simulink model "MSBR_Plant"  (R2021b)
settings: Solver=ode45  StartTime=0.0  StopTime=sim_time  MaxStep=ts_max  RelTol=1e-4
values from neighbouring files (symbols this model uses):
  a_1 = 8.7292e-2/wilson_ratio    (= 0.0087292)    [Whole_Plant_Cool_Pump_Accident_script.m]    (also in Whole_Plant_Fert_Pump_Accident_script.m; Whole_Plant_Fuel_Pump_Accident.m; Whole_Plant_Fuel_Pump_Accident_script.m; Whole_Plant_Reactivity_Accident.m)
  a_2 = 7.3787e-4/wilson_ratio    (= 7.3787e-05)    [Whole_Plant_Cool_Pump_Accident_script.m]    (also in Whole_Plant_Fert_Pump_Accident_script.m; Whole_Plant_Fuel_Pump_Accident.m; Whole_Plant_Fuel_Pump_Accident_script.m; Whole_Plant_Reactivity_Accident.m)
  a_b = 1.656e-5    (= 1.656e-05)    [Whole_Plant_Cool_Pump_Accident_script.m]    (also in Whole_Plant_Fert_Pump_Accident_script.m; Whole_Plant_Fuel_Pump_Accident.m; Whole_Plant_Fuel_Pump_Accident_script.m; Whole_Plant_Reactivity_Accident.m)
  a_f = -8.172e-5    (= -8.172e-05)    [Whole_Plant_Cool_Pump_Accident_script.m]    (also in Whole_Plant_Fert_Pump_Accident_script.m; Whole_Plant_Fuel_Pump_Accident.m; Whole_Plant_Fuel_Pump_Accident_script.m; Whole_Plant_Reactivity_Accident.m)
  a_g = 2.016e-5    (= 2.016e-05)    [Whole_Plant_Cool_Pump_Accident_script.m]    (also in Whole_Plant_Fert_Pump_Accident_script.m; Whole_Plant_Fuel_Pump_Accident.m; Whole_Plant_Fuel_Pump_Accident_script.m; Whole_Plant_Reactivity_Accident.m)
  A_s = pi()*((D_OTSG_i^2)/4) - A_w_OTSG - A_p_OTSG    [Whole_Plant_Cool_Pump_Accident_script.m]    (also in Whole_Plant_Fert_Pump_Accident_script.m; Whole_Plant_Fuel_Pump_Accident.m; Whole_Plant_Fuel_Pump_Accident_script.m; Whole_Plant_Reactivity_Accident.m)
  alpha_co = 316.2    [Whole_Plant_Cool_Pump_Accident_script.m]    (also in Whole_Plant_Fert_Pump_Accident_script.m; Whole_Plant_Fuel_Pump_Accident.m; Whole_Plant_Fuel_Pump_Accident_script.m; Whole_Plant_Reactivity_Accident.m)
  beta = [2.290e-04, 8.320e-04, 7.100e-04, 8.520e-04, 1.710e-04, 1.020e-04]    [Whole_Plant_Cool_Pump_Accident_script.m]    (also in Whole_Plant_Fert_Pump_Accident_script.m; Whole_Plant_Fuel_Pump_Accident.m; Whole_Plant_Fuel_Pump_Accident_script.m; Whole_Plant_Reactivity_Accident.m)
  beta_co = 68.0958    [Whole_Plant_Cool_Pump_Accident_script.m]    (also in Whole_Plant_Fert_Pump_Accident_script.m; Whole_Plant_Fuel_Pump_Accident.m; Whole_Plant_Fuel_Pump_Accident_script.m; Whole_Plant_Reactivity_Accident.m)
  beta_t = sum(beta)    [Whole_Plant_Cool_Pump_Accident_script.m]    (also in Whole_Plant_Fert_Pump_Accident_script.m; Whole_Plant_Fuel_Pump_Accident.m; Whole_Plant_Fuel_Pump_Accident_script.m; Whole_Plant_Reactivity_Accident.m)
  C_nc_X_A_nc = 12.8    [Whole_Plant_Cool_Pump_Accident_script.m]    (also in Whole_Plant_Fert_Pump_Accident_script.m; Whole_Plant_Fuel_Pump_Accident.m; Whole_Plant_Fuel_Pump_Accident_script.m; Whole_Plant_Reactivity_Accident.m)
  C_pcw = 0.0042    [Whole_Plant_Cool_Pump_Accident_script.m]    (also in Whole_Plant_Fert_Pump_Accident_script.m; Whole_Plant_Fuel_Pump_Accident.m; Whole_Plant_Fuel_Pump_Accident_script.m; Whole_Plant_Reactivity_Accident.m)
  C_rh_X_A_rh = 33    [Whole_Plant_Cool_Pump_Accident_script.m]    (also in Whole_Plant_Fert_Pump_Accident_script.m; Whole_Plant_Fuel_Pump_Accident.m; Whole_Plant_Fuel_Pump_Accident_script.m; Whole_Plant_Reactivity_Accident.m)
  C_v = 0.84    [Whole_Plant_Cool_Pump_Accident_script.m]    (also in Whole_Plant_Fert_Pump_Accident_script.m; Whole_Plant_Fuel_Pump_Accident.m; Whole_Plant_Fuel_Pump_Accident_script.m; Whole_Plant_Reactivity_Accident.m)
  ce1 = 1.2471e-07    [Whole_Plant_Cool_Pump_Accident_script.m]    (also in Whole_Plant_Fert_Pump_Accident_script.m; Whole_Plant_Fuel_Pump_Accident.m; Whole_Plant_Fuel_Pump_Accident_script.m; Whole_Plant_Reactivity_Accident.m)
  ce2 = 5.3816e-14    [Whole_Plant_Cool_Pump_Accident_script.m]    (also in Whole_Plant_Fert_Pump_Accident_script.m; Whole_Plant_Fuel_Pump_Accident.m; Whole_Plant_Fuel_Pump_Accident_script.m; Whole_Plant_Reactivity_Accident.m)
  ce3 = 3.3721e-08    [Whole_Plant_Cool_Pump_Accident_script.m]    (also in Whole_Plant_Fert_Pump_Accident_script.m; Whole_Plant_Fuel_Pump_Accident.m; Whole_Plant_Fuel_Pump_Accident_script.m; Whole_Plant_Reactivity_Accident.m)
  Cp_fw = XSteam('Cp_pT',P_set*10,T_fw)/1000    [Whole_Plant_Cool_Pump_Accident_script.m]    (also in Whole_Plant_Fert_Pump_Accident_script.m; Whole_Plant_Fuel_Pump_Accident.m; Whole_Plant_Fuel_Pump_Accident_script.m; Whole_Plant_Reactivity_Accident.m)
  Cp_p = Cp_sec    (= 0.001716588)    [Whole_Plant_Cool_Pump_Accident_script.m]    (also in Whole_Plant_Fert_Pump_Accident_script.m; Whole_Plant_Fuel_Pump_Accident.m; Whole_Plant_Fuel_Pump_Accident_script.m; Whole_Plant_Reactivity_Accident.m)
  Cp_rh = 0.0021520    (= 0.002152)    [Whole_Plant_Cool_Pump_Accident_script.m]    (also in Whole_Plant_Fert_Pump_Accident_script.m; Whole_Plant_Fuel_Pump_Accident.m; Whole_Plant_Fuel_Pump_Accident_script.m; Whole_Plant_Reactivity_Accident.m)
  Cp_s = XSteam('Cp_pT',P_s*10,T_s)/1000    [Whole_Plant_Cool_Pump_Accident_script.m]    (also in Whole_Plant_Fert_Pump_Accident_script.m; Whole_Plant_Fuel_Pump_Accident.m; Whole_Plant_Fuel_Pump_Accident_script.m; Whole_Plant_Reactivity_Accident.m)
  Cp_sc = XSteam('Cp_pT',P_set*10,T_sc2)/1000    [Whole_Plant_Cool_Pump_Accident_script.m]    (also in Whole_Plant_Fert_Pump_Accident_script.m; Whole_Plant_Fuel_Pump_Accident.m; Whole_Plant_Fuel_Pump_Accident_script.m; Whole_Plant_Reactivity_Accident.m)
  Cp_w = 468.992e-6    (= 0.000468992)    [Whole_Plant_Cool_Pump_Accident_script.m]    (also in Whole_Plant_Fert_Pump_Accident_script.m; Whole_Plant_Fuel_Pump_Accident.m; Whole_Plant_Fuel_Pump_Accident_script.m; Whole_Plant_Reactivity_Accident.m)
  D_it = D_ot-2*T_th    (= 0.014147)    [Whole_Plant_Cool_Pump_Accident_script.m]    (also in Whole_Plant_Fert_Pump_Accident_script.m; Whole_Plant_Fuel_Pump_Accident.m; Whole_Plant_Fuel_Pump_Accident_script.m; Whole_Plant_Reactivity_Accident.m)
  D_ot = 0.015875    [Whole_Plant_Cool_Pump_Accident_script.m]    (also in Whole_Plant_Fert_Pump_Accident_script.m; Whole_Plant_Fuel_Pump_Accident.m; Whole_Plant_Fuel_Pump_Accident_script.m; Whole_Plant_Reactivity_Accident.m)
  dHs_dPs = c(1)    [Whole_Plant_Cool_Pump_Accident_script.m]    (also in Whole_Plant_Fert_Pump_Accident_script.m; Whole_Plant_Fuel_Pump_Accident.m; Whole_Plant_Fuel_Pump_Accident_script.m; Whole_Plant_Reactivity_Accident.m)
  eta_hp_isen = 0.861    [Whole_Plant_Cool_Pump_Accident_script.m]    (also in Whole_Plant_Fert_Pump_Accident_script.m; Whole_Plant_Fuel_Pump_Accident.m; Whole_Plant_Fuel_Pump_Accident_script.m; Whole_Plant_Reactivity_Accident.m)
  eta_lp_isen = 0.861    [Whole_Plant_Cool_Pump_Accident_script.m]    (also in Whole_Plant_Fert_Pump_Accident_script.m; Whole_Plant_Fuel_Pump_Accident.m; Whole_Plant_Fuel_Pump_Accident_script.m; Whole_Plant_Reactivity_Accident.m)
  gamma_I = 5.1135e-2    (= 0.051135)    [Whole_Plant_Cool_Pump_Accident_script.m]    (also in Whole_Plant_Fert_Pump_Accident_script.m; Whole_Plant_Fuel_Pump_Accident.m; Whole_Plant_Fuel_Pump_Accident_script.m; Whole_Plant_Reactivity_Accident.m)
  gamma_Xe = 1.1628e-2    (= 0.011628)    [Whole_Plant_Cool_Pump_Accident_script.m]    (also in Whole_Plant_Fert_Pump_Accident_script.m; Whole_Plant_Fuel_Pump_Accident.m; Whole_Plant_Fuel_Pump_Accident_script.m; Whole_Plant_Reactivity_Accident.m)
  H_co0 = 0.149    [Whole_Plant_Cool_Pump_Accident_script.m]    (also in Whole_Plant_Fert_Pump_Accident_script.m; Whole_Plant_Fuel_Pump_Accident.m; Whole_Plant_Fuel_Pump_Accident_script.m; Whole_Plant_Reactivity_Accident.m)
  H_f_co0 = 0.149    [Whole_Plant_Cool_Pump_Accident_script.m]    (also in Whole_Plant_Fert_Pump_Accident_script.m; Whole_Plant_Fuel_Pump_Accident.m; Whole_Plant_Fuel_Pump_Accident_script.m; Whole_Plant_Reactivity_Accident.m)
  H_fg_co0 = 2.35    [Whole_Plant_Cool_Pump_Accident_script.m]    (also in Whole_Plant_Fert_Pump_Accident_script.m; Whole_Plant_Fuel_Pump_Accident.m; Whole_Plant_Fuel_Pump_Accident_script.m; Whole_Plant_Reactivity_Accident.m)
  H_fgrh0 = (XSteam('hV_p', P_s*1e1) - XSteam('hL_p', P_s*1e1))/1e3    [Whole_Plant_Cool_Pump_Accident_script.m]    (also in Whole_Plant_Fert_Pump_Accident_script.m; Whole_Plant_Fuel_Pump_Accident.m; Whole_Plant_Fuel_Pump_Accident_script.m; Whole_Plant_Reactivity_Accident.m)
  H_frh0 = XSteam('hL_p', P_s*1e1)/1e3    [Whole_Plant_Cool_Pump_Accident_script.m]    (also in Whole_Plant_Fert_Pump_Accident_script.m; Whole_Plant_Fuel_Pump_Accident.m; Whole_Plant_Fuel_Pump_Accident_script.m; Whole_Plant_Reactivity_Accident.m)
  h_fwh1 = 0.5927    [Whole_Plant_Cool_Pump_Accident_script.m]    (also in Whole_Plant_Fert_Pump_Accident_script.m; Whole_Plant_Fuel_Pump_Accident.m; Whole_Plant_Fuel_Pump_Accident_script.m; Whole_Plant_Reactivity_Accident.m)
  H_fwh10 = 0.46009    [Whole_Plant_Cool_Pump_Accident_script.m]    (also in Whole_Plant_Fert_Pump_Accident_script.m; Whole_Plant_Fuel_Pump_Accident.m; Whole_Plant_Fuel_Pump_Accident_script.m; Whole_Plant_Reactivity_Accident.m)
  h_fwh2 = 1.230803    [Whole_Plant_Cool_Pump_Accident_script.m]    (also in Whole_Plant_Fert_Pump_Accident_script.m; Whole_Plant_Fuel_Pump_Accident.m; Whole_Plant_Fuel_Pump_Accident_script.m; Whole_Plant_Reactivity_Accident.m)
  H_fwh20 = 0.6784    [Whole_Plant_Cool_Pump_Accident_script.m]    (also in Whole_Plant_Fert_Pump_Accident_script.m; Whole_Plant_Fuel_Pump_Accident.m; Whole_Plant_Fuel_Pump_Accident_script.m; Whole_Plant_Reactivity_Accident.m)
  H_grh0 = 2.8029    [Whole_Plant_Cool_Pump_Accident_script.m]    (also in Whole_Plant_Fert_Pump_Accident_script.m; Whole_Plant_Fuel_Pump_Accident.m; Whole_Plant_Fuel_Pump_Accident_script.m; Whole_Plant_Reactivity_Accident.m)
  H_hp_isen0 = 2.5111    [Whole_Plant_Cool_Pump_Accident_script.m]    (also in Whole_Plant_Fert_Pump_Accident_script.m; Whole_Plant_Fuel_Pump_Accident.m; Whole_Plant_Fuel_Pump_Accident_script.m; Whole_Plant_Reactivity_Accident.m)
  H_hpt_out = 2.6201    [Whole_Plant_Cool_Pump_Accident_script.m]    (also in Whole_Plant_Fert_Pump_Accident_script.m; Whole_Plant_Fuel_Pump_Accident.m; Whole_Plant_Fuel_Pump_Accident_script.m; Whole_Plant_Reactivity_Accident.m)
  H_lp_isen = 958.4*1054.35e-6/0.45359237    (= 2.22774699671)    [Whole_Plant_Cool_Pump_Accident_script.m]    (also in Whole_Plant_Fert_Pump_Accident_script.m; Whole_Plant_Fuel_Pump_Accident.m; Whole_Plant_Fuel_Pump_Accident_script.m; Whole_Plant_Reactivity_Accident.m)
  H_lpt_out = 2.3089    [Whole_Plant_Cool_Pump_Accident_script.m]    (also in Whole_Plant_Fert_Pump_Accident_script.m; Whole_Plant_Fuel_Pump_Accident.m; Whole_Plant_Fuel_Pump_Accident_script.m; Whole_Plant_Reactivity_Accident.m)
  H_nc = XSteam('h_pT', P_s*10, T_s)/1000    [Whole_Plant_Cool_Pump_Accident_script.m]    (also in Whole_Plant_Fert_Pump_Accident_script.m; Whole_Plant_Fuel_Pump_Accident.m; Whole_Plant_Fuel_Pump_Accident_script.m; Whole_Plant_Reactivity_Accident.m)
  h_pw = h_s    (= 0.02555)    [Whole_Plant_Cool_Pump_Accident_script.m]    (also in Whole_Plant_Fert_Pump_Accident_script.m; Whole_Plant_Fuel_Pump_Accident.m; Whole_Plant_Fuel_Pump_Accident_script.m; Whole_Plant_Reactivity_Accident.m)
  H_rh = 2.8115    [Whole_Plant_Cool_Pump_Accident_script.m]    (also in Whole_Plant_Fert_Pump_Accident_script.m; Whole_Plant_Fuel_Pump_Accident.m; Whole_Plant_Fuel_Pump_Accident_script.m; Whole_Plant_Reactivity_Accident.m)
  h_wb = 13349.334646671E-6    (= 0.0133493346467)    [Whole_Plant_Cool_Pump_Accident_script.m]    (also in Whole_Plant_Fert_Pump_Accident_script.m; Whole_Plant_Fuel_Pump_Accident.m; Whole_Plant_Fuel_Pump_Accident_script.m; Whole_Plant_Reactivity_Accident.m)
  h_ws = 5732.378387768E-6    (= 0.00573237838777)    [Whole_Plant_Cool_Pump_Accident_script.m]    (also in Whole_Plant_Fert_Pump_Accident_script.m; Whole_Plant_Fuel_Pump_Accident.m; Whole_Plant_Fuel_Pump_Accident_script.m; Whole_Plant_Reactivity_Accident.m)
  h_wsc = 8385.005556375E-6    (= 0.00838500555638)    [Whole_Plant_Cool_Pump_Accident_script.m]    (also in Whole_Plant_Fert_Pump_Accident_script.m; Whole_Plant_Fuel_Pump_Accident.m; Whole_Plant_Fuel_Pump_Accident_script.m; Whole_Plant_Reactivity_Accident.m)
  hA_bg = A_fert*h_bg    (= 2.76411813627)    [Whole_Plant_Cool_Pump_Accident_script.m]    (also in Whole_Plant_Fert_Pump_Accident_script.m; Whole_Plant_Fuel_Pump_Accident.m; Whole_Plant_Fuel_Pump_Accident_script.m; Whole_Plant_Reactivity_Accident.m)
  hA_co0 = 140    [Whole_Plant_Cool_Pump_Accident_script.m]    (also in Whole_Plant_Fert_Pump_Accident_script.m; Whole_Plant_Fuel_Pump_Accident.m; Whole_Plant_Fuel_Pump_Accident_script.m; Whole_Plant_Reactivity_Accident.m)
  hA_fg_dn = h_fg*A_fuel_down    [Whole_Plant_Cool_Pump_Accident_script.m]    (also in Whole_Plant_Fert_Pump_Accident_script.m; Whole_Plant_Fuel_Pump_Accident.m; Whole_Plant_Fuel_Pump_Accident_script.m; Whole_Plant_Reactivity_Accident.m)
  hA_fg_up = h_fg*A_fuel_up    [Whole_Plant_Cool_Pump_Accident_script.m]    (also in Whole_Plant_Fert_Pump_Accident_script.m; Whole_Plant_Fuel_Pump_Accident.m; Whole_Plant_Fuel_Pump_Accident_script.m; Whole_Plant_Reactivity_Accident.m)
  hA_p_bhx1 = [h_pb*A_pbhx/2,h_pb*A_pbhx/2]    [Whole_Plant_Cool_Pump_Accident_script.m]    (also in Whole_Plant_Fert_Pump_Accident_script.m; Whole_Plant_Fuel_Pump_Accident.m; Whole_Plant_Fuel_Pump_Accident_script.m; Whole_Plant_Reactivity_Accident.m)
  hA_p_bhx2 = hA_p_bhx1    [Whole_Plant_Cool_Pump_Accident_script.m]    (also in Whole_Plant_Fert_Pump_Accident_script.m; Whole_Plant_Fuel_Pump_Accident.m; Whole_Plant_Fuel_Pump_Accident_script.m; Whole_Plant_Reactivity_Accident.m)
  hA_p_bhx3 = hA_p_bhx1    [Whole_Plant_Cool_Pump_Accident_script.m]    (also in Whole_Plant_Fert_Pump_Accident_script.m; Whole_Plant_Fuel_Pump_Accident.m; Whole_Plant_Fuel_Pump_Accident_script.m; Whole_Plant_Reactivity_Accident.m)
  hA_p_bhx4 = hA_p_bhx1    [Whole_Plant_Cool_Pump_Accident_script.m]    (also in Whole_Plant_Fert_Pump_Accident_script.m; Whole_Plant_Fuel_Pump_Accident.m; Whole_Plant_Fuel_Pump_Accident_script.m; Whole_Plant_Reactivity_Accident.m)
  hA_p_fhx1 = [h_p*A_pfhx_dn/2,h_p*A_pfhx_dn/2,h_p*A_pfhx_up/2,h_p*A_pfhx_up/2]    [Whole_Plant_Cool_Pump_Accident_script.m]    (also in Whole_Plant_Fert_Pump_Accident_script.m; Whole_Plant_Fuel_Pump_Accident.m; Whole_Plant_Fuel_Pump_Accident_script.m; Whole_Plant_Reactivity_Accident.m)
  hA_p_fhx2 = hA_p_fhx1    [Whole_Plant_Cool_Pump_Accident_script.m]    (also in Whole_Plant_Fert_Pump_Accident_script.m; Whole_Plant_Fuel_Pump_Accident.m; Whole_Plant_Fuel_Pump_Accident_script.m; Whole_Plant_Reactivity_Accident.m)
  hA_p_fhx3 = hA_p_fhx1    [Whole_Plant_Cool_Pump_Accident_script.m]    (also in Whole_Plant_Fert_Pump_Accident_script.m; Whole_Plant_Fuel_Pump_Accident.m; Whole_Plant_Fuel_Pump_Accident_script.m; Whole_Plant_Reactivity_Accident.m)
  hA_p_fhx4 = hA_p_fhx1    [Whole_Plant_Cool_Pump_Accident_script.m]    (also in Whole_Plant_Fert_Pump_Accident_script.m; Whole_Plant_Fuel_Pump_Accident.m; Whole_Plant_Fuel_Pump_Accident_script.m; Whole_Plant_Reactivity_Accident.m)
  hA_s_bhx1 = [h_sb*A_sbhx/2,h_sb*A_sbhx/2]    [Whole_Plant_Cool_Pump_Accident_script.m]    (also in Whole_Plant_Fert_Pump_Accident_script.m; Whole_Plant_Fuel_Pump_Accident.m; Whole_Plant_Fuel_Pump_Accident_script.m; Whole_Plant_Reactivity_Accident.m)
  hA_s_bhx2 = hA_s_bhx1    [Whole_Plant_Cool_Pump_Accident_script.m]    (also in Whole_Plant_Fert_Pump_Accident_script.m; Whole_Plant_Fuel_Pump_Accident.m; Whole_Plant_Fuel_Pump_Accident_script.m; Whole_Plant_Reactivity_Accident.m)
  hA_s_bhx3 = hA_s_bhx1    [Whole_Plant_Cool_Pump_Accident_script.m]    (also in Whole_Plant_Fert_Pump_Accident_script.m; Whole_Plant_Fuel_Pump_Accident.m; Whole_Plant_Fuel_Pump_Accident_script.m; Whole_Plant_Reactivity_Accident.m)
  hA_s_bhx4 = hA_s_bhx1    [Whole_Plant_Cool_Pump_Accident_script.m]    (also in Whole_Plant_Fert_Pump_Accident_script.m; Whole_Plant_Fuel_Pump_Accident.m; Whole_Plant_Fuel_Pump_Accident_script.m; Whole_Plant_Reactivity_Accident.m)
  hA_s_fhx1 = [h_s*A_sfhx_up/2,h_s*A_sfhx_up/2,h_s*A_sfhx_dn/2,h_s*A_sfhx_dn/2]    [Whole_Plant_Cool_Pump_Accident_script.m]    (also in Whole_Plant_Fert_Pump_Accident_script.m; Whole_Plant_Fuel_Pump_Accident.m; Whole_Plant_Fuel_Pump_Accident_script.m; Whole_Plant_Reactivity_Accident.m)
  hA_s_fhx2 = hA_s_fhx1    [Whole_Plant_Cool_Pump_Accident_script.m]    (also in Whole_Plant_Fert_Pump_Accident_script.m; Whole_Plant_Fuel_Pump_Accident.m; Whole_Plant_Fuel_Pump_Accident_script.m; Whole_Plant_Reactivity_Accident.m)
  hA_s_fhx3 = hA_s_fhx1    [Whole_Plant_Cool_Pump_Accident_script.m]    (also in Whole_Plant_Fert_Pump_Accident_script.m; Whole_Plant_Fuel_Pump_Accident.m; Whole_Plant_Fuel_Pump_Accident_script.m; Whole_Plant_Reactivity_Accident.m)
  hA_s_fhx4 = hA_s_fhx1    [Whole_Plant_Cool_Pump_Accident_script.m]    (also in Whole_Plant_Fert_Pump_Accident_script.m; Whole_Plant_Fuel_Pump_Accident.m; Whole_Plant_Fuel_Pump_Accident_script.m; Whole_Plant_Reactivity_Accident.m)
  I_0 = gamma_I*Sigma_f_msbr*phi_0/lam_I    (= 1.30000734126e+17)    [Whole_Plant_Cool_Pump_Accident_script.m]    (also in Whole_Plant_Fert_Pump_Accident_script.m; Whole_Plant_Fuel_Pump_Accident.m; Whole_Plant_Fuel_Pump_Accident_script.m; Whole_Plant_Reactivity_Accident.m)
  k_1 = 0.5    [Whole_Plant_Cool_Pump_Accident_script.m]    (also in Whole_Plant_Fert_Pump_Accident_script.m; Whole_Plant_Fuel_Pump_Accident.m; Whole_Plant_Fuel_Pump_Accident_script.m; Whole_Plant_Reactivity_Accident.m)
  K_1 = e(1)    [Whole_Plant_Cool_Pump_Accident_script.m]    (also in Whole_Plant_Fert_Pump_Accident_script.m; Whole_Plant_Fuel_Pump_Accident.m; Whole_Plant_Fuel_Pump_Accident_script.m; Whole_Plant_Reactivity_Accident.m)
  k_1b = 0.5    [Whole_Plant_Cool_Pump_Accident_script.m]    (also in Whole_Plant_Fert_Pump_Accident_script.m; Whole_Plant_Fuel_Pump_Accident.m; Whole_Plant_Fuel_Pump_Accident_script.m; Whole_Plant_Reactivity_Accident.m)
  k_2 = 0.5    [Whole_Plant_Cool_Pump_Accident_script.m]    (also in Whole_Plant_Fert_Pump_Accident_script.m; Whole_Plant_Fuel_Pump_Accident.m; Whole_Plant_Fuel_Pump_Accident_script.m; Whole_Plant_Reactivity_Accident.m)
  k_2b = 0.5    [Whole_Plant_Cool_Pump_Accident_script.m]    (also in Whole_Plant_Fert_Pump_Accident_script.m; Whole_Plant_Fuel_Pump_Accident.m; Whole_Plant_Fuel_Pump_Accident_script.m; Whole_Plant_Reactivity_Accident.m)
  k_3 = 0.5    [Whole_Plant_Cool_Pump_Accident_script.m]    (also in Whole_Plant_Fert_Pump_Accident_script.m; Whole_Plant_Fuel_Pump_Accident.m; Whole_Plant_Fuel_Pump_Accident_script.m; Whole_Plant_Reactivity_Accident.m)
  k_4 = 0.5    [Whole_Plant_Cool_Pump_Accident_script.m]    (also in Whole_Plant_Fert_Pump_Accident_script.m; Whole_Plant_Fuel_Pump_Accident.m; Whole_Plant_Fuel_Pump_Accident_script.m; Whole_Plant_Reactivity_Accident.m)
  K_4 = b(1)    [Whole_Plant_Cool_Pump_Accident_script.m]    (also in Whole_Plant_Fert_Pump_Accident_script.m; Whole_Plant_Fuel_Pump_Accident.m; Whole_Plant_Fuel_Pump_Accident_script.m; Whole_Plant_Reactivity_Accident.m)
  K_5 = a(1)    [Whole_Plant_Cool_Pump_Accident_script.m]    (also in Whole_Plant_Fert_Pump_Accident_script.m; Whole_Plant_Fuel_Pump_Accident.m; Whole_Plant_Fuel_Pump_Accident_script.m; Whole_Plant_Reactivity_Accident.m)
  K_b = d(1)    [Whole_Plant_Cool_Pump_Accident_script.m]    (also in Whole_Plant_Fert_Pump_Accident_script.m; Whole_Plant_Fuel_Pump_Accident.m; Whole_Plant_Fuel_Pump_Accident_script.m; Whole_Plant_Reactivity_Accident.m)
  k_b1 = (K_B/2)/K    (= 0.0089463103122)    [Whole_Plant_Cool_Pump_Accident_script.m]    (also in Whole_Plant_Fert_Pump_Accident_script.m; Whole_Plant_Fuel_Pump_Accident.m; Whole_Plant_Fuel_Pump_Accident_script.m; Whole_Plant_Reactivity_Accident.m)
  k_b2 = k_b1    (= 0.0089463103122)    [Whole_Plant_Cool_Pump_Accident_script.m]    (also in Whole_Plant_Fert_Pump_Accident_script.m; Whole_Plant_Fuel_Pump_Accident.m; Whole_Plant_Fuel_Pump_Accident_script.m; Whole_Plant_Reactivity_Accident.m)
  K_bhp = 0.1634    [Whole_Plant_Cool_Pump_Accident_script.m]    (also in Whole_Plant_Fert_Pump_Accident_script.m; Whole_Plant_Fuel_Pump_Accident.m; Whole_Plant_Fuel_Pump_Accident_script.m; Whole_Plant_Reactivity_Accident.m)
  K_blp = 0.2174    [Whole_Plant_Cool_Pump_Accident_script.m]    (also in Whole_Plant_Fert_Pump_Accident_script.m; Whole_Plant_Fuel_Pump_Accident.m; Whole_Plant_Fuel_Pump_Accident_script.m; Whole_Plant_Reactivity_Accident.m)
  k_f1 = ((1 - K_G - K_B - K_Ba)/4)/K    (= 0.226055463576)    [Whole_Plant_Cool_Pump_Accident_script.m]    (also in Whole_Plant_Fert_Pump_Accident_script.m; Whole_Plant_Fuel_Pump_Accident.m; Whole_Plant_Fuel_Pump_Accident_script.m; Whole_Plant_Reactivity_Accident.m)
  k_f2 = k_f1    (= 0.226055463576)    [Whole_Plant_Cool_Pump_Accident_script.m]    (also in Whole_Plant_Fert_Pump_Accident_script.m; Whole_Plant_Fuel_Pump_Accident.m; Whole_Plant_Fuel_Pump_Accident_script.m; Whole_Plant_Reactivity_Accident.m)
  k_f3 = k_f1    (= 0.226055463576)    [Whole_Plant_Cool_Pump_Accident_script.m]    (also in Whole_Plant_Fert_Pump_Accident_script.m; Whole_Plant_Fuel_Pump_Accident.m; Whole_Plant_Fuel_Pump_Accident_script.m; Whole_Plant_Reactivity_Accident.m)
  k_f4 = k_f1    (= 0.226055463576)    [Whole_Plant_Cool_Pump_Accident_script.m]    (also in Whole_Plant_Fert_Pump_Accident_script.m; Whole_Plant_Fuel_Pump_Accident.m; Whole_Plant_Fuel_Pump_Accident_script.m; Whole_Plant_Reactivity_Accident.m)
  k_g1 = ((K_G*K_fuel)/2)/K    (= 0.0346590586566)    [Whole_Plant_Cool_Pump_Accident_script.m]    (also in Whole_Plant_Fert_Pump_Accident_script.m; Whole_Plant_Fuel_Pump_Accident.m; Whole_Plant_Fuel_Pump_Accident_script.m; Whole_Plant_Reactivity_Accident.m)
  k_g2 = k_g1    (= 0.0346590586566)    [Whole_Plant_Cool_Pump_Accident_script.m]    (also in Whole_Plant_Fert_Pump_Accident_script.m; Whole_Plant_Fuel_Pump_Accident.m; Whole_Plant_Fuel_Pump_Accident_script.m; Whole_Plant_Reactivity_Accident.m)
  k_g3 = (K_G*(1-K_fuel))/K    (= 0.00856740775781)    [Whole_Plant_Cool_Pump_Accident_script.m]    (also in Whole_Plant_Fert_Pump_Accident_script.m; Whole_Plant_Fuel_Pump_Accident.m; Whole_Plant_Fuel_Pump_Accident_script.m; Whole_Plant_Reactivity_Accident.m)
  K_sc = f(1)    [Whole_Plant_Cool_Pump_Accident_script.m]    (also in Whole_Plant_Fert_Pump_Accident_script.m; Whole_Plant_Fuel_Pump_Accident.m; Whole_Plant_Fuel_Pump_Accident_script.m; Whole_Plant_Reactivity_Accident.m)
  L = 22.0    (= 22)    [Whole_Plant_Cool_Pump_Accident_script.m]    (also in Whole_Plant_Fert_Pump_Accident_script.m; Whole_Plant_Fuel_Pump_Accident.m; Whole_Plant_Fuel_Pump_Accident_script.m; Whole_Plant_Reactivity_Accident.m)
  L_b = 1.9    [Whole_Plant_Cool_Pump_Accident_script.m]    (also in Whole_Plant_Fert_Pump_Accident_script.m; Whole_Plant_Fuel_Pump_Accident.m; Whole_Plant_Fuel_Pump_Accident_script.m; Whole_Plant_Reactivity_Accident.m)
  L_s = 16.53    [Whole_Plant_Cool_Pump_Accident_script.m]    (also in Whole_Plant_Fert_Pump_Accident_script.m; Whole_Plant_Fuel_Pump_Accident.m; Whole_Plant_Fuel_Pump_Accident_script.m; Whole_Plant_Reactivity_Accident.m)
  L_sc = L-L_b-L_s    (= 3.57)    [Whole_Plant_Cool_Pump_Accident_script.m]    (also in Whole_Plant_Fert_Pump_Accident_script.m; Whole_Plant_Fuel_Pump_Accident.m; Whole_Plant_Fuel_Pump_Accident_script.m; Whole_Plant_Reactivity_Accident.m)
  Lam = 3.3e-4    (= 0.00033)    [Whole_Plant_Cool_Pump_Accident_script.m]    (also in Whole_Plant_Fert_Pump_Accident_script.m; Whole_Plant_Fuel_Pump_Accident.m; Whole_Plant_Fuel_Pump_Accident_script.m; Whole_Plant_Reactivity_Accident.m)
  lam = [1.260e-02, 3.370e-02, 1.390e-01, 3.250e-01, 1.130e+00, 2.500e+00]    [Whole_Plant_Cool_Pump_Accident_script.m]    (also in Whole_Plant_Fert_Pump_Accident_script.m; Whole_Plant_Fuel_Pump_Accident.m; Whole_Plant_Fuel_Pump_Accident_script.m; Whole_Plant_Reactivity_Accident.m)
  lam_bubl = 2.0e-2    (= 0.02)    [Whole_Plant_Cool_Pump_Accident_script.m]    (also in Whole_Plant_Fert_Pump_Accident_script.m; Whole_Plant_Fuel_Pump_Accident.m; Whole_Plant_Fuel_Pump_Accident_script.m; Whole_Plant_Reactivity_Accident.m)
  lam_I = 2.875e-5    (= 2.875e-05)    [Whole_Plant_Cool_Pump_Accident_script.m]    (also in Whole_Plant_Fert_Pump_Accident_script.m; Whole_Plant_Fuel_Pump_Accident.m; Whole_Plant_Fuel_Pump_Accident_script.m; Whole_Plant_Reactivity_Accident.m)
  lam_Xe = 2.0916e-5    (= 2.0916e-05)    [Whole_Plant_Cool_Pump_Accident_script.m]    (also in Whole_Plant_Fert_Pump_Accident_script.m; Whole_Plant_Fuel_Pump_Accident.m; Whole_Plant_Fuel_Pump_Accident_script.m; Whole_Plant_Reactivity_Accident.m)
  m_bm = (W_b1+W_b2+W_b3+W_b4)*time_mixb    (= 2167.1636)    [Whole_Plant_Cool_Pump_Accident_script.m]    (also in Whole_Plant_Fert_Pump_Accident_script.m; Whole_Plant_Fuel_Pump_Accident.m; Whole_Plant_Fuel_Pump_Accident_script.m; Whole_Plant_Reactivity_Accident.m)
  M_cw = 65000    [Whole_Plant_Cool_Pump_Accident_script.m]    (also in Whole_Plant_Fert_Pump_Accident_script.m; Whole_Plant_Fuel_Pump_Accident.m; Whole_Plant_Fuel_Pump_Accident_script.m; Whole_Plant_Reactivity_Accident.m)
  m_fm = (W_f1+W_f2+W_f3+W_f4)*time_mixf    (= 5443.108)    [Whole_Plant_Cool_Pump_Accident_script.m]    (also in Whole_Plant_Fert_Pump_Accident_script.m; Whole_Plant_Fuel_Pump_Accident.m; Whole_Plant_Fuel_Pump_Accident_script.m; Whole_Plant_Reactivity_Accident.m)
  M_hw0 = 10000    [Whole_Plant_Cool_Pump_Accident_script.m]    (also in Whole_Plant_Fert_Pump_Accident_script.m; Whole_Plant_Fuel_Pump_Accident.m; Whole_Plant_Fuel_Pump_Accident_script.m; Whole_Plant_Reactivity_Accident.m)
  m_sm = (W_s1+W_s2+W_s3+W_s4)*time_mixs    (= 8467.056)    [Whole_Plant_Cool_Pump_Accident_script.m]    (also in Whole_Plant_Fert_Pump_Accident_script.m; Whole_Plant_Fuel_Pump_Accident.m; Whole_Plant_Fuel_Pump_Accident_script.m; Whole_Plant_Reactivity_Accident.m)
  M_stm = 0.018    [Whole_Plant_Cool_Pump_Accident_script.m]    (also in Whole_Plant_Fert_Pump_Accident_script.m; Whole_Plant_Fuel_Pump_Accident.m; Whole_Plant_Fuel_Pump_Accident_script.m; Whole_Plant_Reactivity_Accident.m)
  mcp_b1 = mass_bn*Cp_b    (= 4.17494922705)    [Whole_Plant_Cool_Pump_Accident_script.m]    (also in Whole_Plant_Fert_Pump_Accident_script.m; Whole_Plant_Fuel_Pump_Accident.m; Whole_Plant_Fuel_Pump_Accident_script.m; Whole_Plant_Reactivity_Accident.m)
  mcp_b2 = mcp_b1    (= 4.17494922705)    [Whole_Plant_Cool_Pump_Accident_script.m]    (also in Whole_Plant_Fert_Pump_Accident_script.m; Whole_Plant_Fuel_Pump_Accident.m; Whole_Plant_Fuel_Pump_Accident_script.m; Whole_Plant_Reactivity_Accident.m)
  mcp_f1 = mass_fn*Cp_f    (= 5.5019469141)    [Whole_Plant_Cool_Pump_Accident_script.m]    (also in Whole_Plant_Fert_Pump_Accident_script.m; Whole_Plant_Fuel_Pump_Accident.m; Whole_Plant_Fuel_Pump_Accident_script.m; Whole_Plant_Reactivity_Accident.m)
  mcp_f2 = mass_fn*Cp_f    (= 5.5019469141)    [Whole_Plant_Cool_Pump_Accident_script.m]    (also in Whole_Plant_Fert_Pump_Accident_script.m; Whole_Plant_Fuel_Pump_Accident.m; Whole_Plant_Fuel_Pump_Accident_script.m; Whole_Plant_Reactivity_Accident.m)
  mcp_f3 = mass_fn*Cp_f    (= 5.5019469141)    [Whole_Plant_Cool_Pump_Accident_script.m]    (also in Whole_Plant_Fert_Pump_Accident_script.m; Whole_Plant_Fuel_Pump_Accident.m; Whole_Plant_Fuel_Pump_Accident_script.m; Whole_Plant_Reactivity_Accident.m)
  mcp_f4 = mass_fn*Cp_f    (= 5.5019469141)    [Whole_Plant_Cool_Pump_Accident_script.m]    (also in Whole_Plant_Fert_Pump_Accident_script.m; Whole_Plant_Fuel_Pump_Accident.m; Whole_Plant_Fuel_Pump_Accident_script.m; Whole_Plant_Reactivity_Accident.m)
  mcp_g1 = (mass_grap*Cp_g)*K_fuel/2    (= 32.9814988203)    [Whole_Plant_Cool_Pump_Accident_script.m]    (also in Whole_Plant_Fert_Pump_Accident_script.m; Whole_Plant_Fuel_Pump_Accident.m; Whole_Plant_Fuel_Pump_Accident_script.m; Whole_Plant_Reactivity_Accident.m)
  mcp_g2 = mcp_g1    (= 32.9814988203)    [Whole_Plant_Cool_Pump_Accident_script.m]    (also in Whole_Plant_Fert_Pump_Accident_script.m; Whole_Plant_Fuel_Pump_Accident.m; Whole_Plant_Fuel_Pump_Accident_script.m; Whole_Plant_Reactivity_Accident.m)
  mcp_g3 = (mass_grap*Cp_g)*(1-K_fuel)    (= 8.15273004546)    [Whole_Plant_Cool_Pump_Accident_script.m]    (also in Whole_Plant_Fert_Pump_Accident_script.m; Whole_Plant_Fuel_Pump_Accident.m; Whole_Plant_Fuel_Pump_Accident_script.m; Whole_Plant_Reactivity_Accident.m)
  mcp_p_bhx1 = mp_bhx1*Cp_b    [Whole_Plant_Cool_Pump_Accident_script.m]    (also in Whole_Plant_Fert_Pump_Accident_script.m; Whole_Plant_Fuel_Pump_Accident.m; Whole_Plant_Fuel_Pump_Accident_script.m; Whole_Plant_Reactivity_Accident.m)
  mcp_p_bhx2 = mp_bhx2*Cp_b    [Whole_Plant_Cool_Pump_Accident_script.m]    (also in Whole_Plant_Fert_Pump_Accident_script.m; Whole_Plant_Fuel_Pump_Accident.m; Whole_Plant_Fuel_Pump_Accident_script.m; Whole_Plant_Reactivity_Accident.m)
  mcp_p_bhx3 = mp_bhx3*Cp_b    [Whole_Plant_Cool_Pump_Accident_script.m]    (also in Whole_Plant_Fert_Pump_Accident_script.m; Whole_Plant_Fuel_Pump_Accident.m; Whole_Plant_Fuel_Pump_Accident_script.m; Whole_Plant_Reactivity_Accident.m)
  ... (+213 more)
undefined symbols (not defined in the file or in its folder): C0, H_con_table, H_convap_table, H_rh_table, H_rh_table1, H_rh_table2, H_rhvap_table, H_s_table, H_table, P_con_table, P_nc_table, P_rh_table, P_rh_table1, pres_table, rho_rh_table, rho_table, SV_nc_table, SVf_nc_table, temp_table
(part 13 of 13)

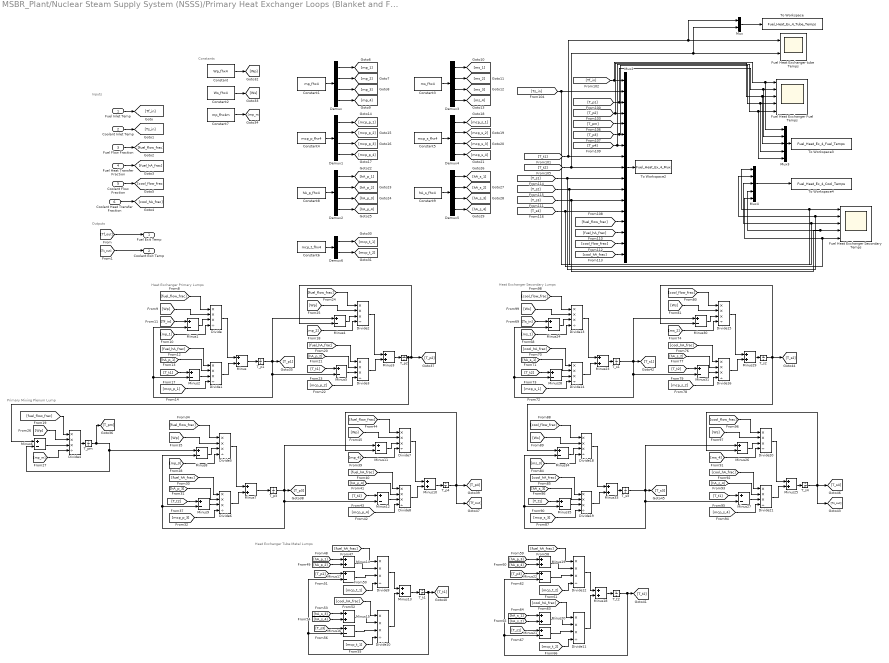
== system MSBR_Plant/Nuclear Steam Supply System (NSSS)/Primary Heat Exchanger Loops (Blanket and Fuel Salt HXs)/HEAT EXCHANGER LOOP 4/Fuel Heat Exchanger Heat Transfer ==
  note: Constants
  note: Primary Mixing Plenum Lump
  note: Heat Exchanger Tube Metal Lumps
  note: Heat Exchanger Primary Lumps
  note: Outputs
  note: Heat Exchanger Secondary Lumps
  note: Inputs
  Fuel Inlet Temp : Inport
  Coolant Inlet Temp : Inport  Port=2
  Fuel Flow Fraction : Inport  Port=3
  Fuel Heat Transfer Fraction : Inport  Port=4
  Coolant Flow Fraction : Inport  Port=5
  Coolant Heat Transfer Fraction : Inport  Port=6
  Constant : Constant  Value=Wp_fhx4
  Constant1 : Constant  Value=mp_fhx4
  Constant2 : Constant  Value=Ws_fhx4
  Constant3 : Constant  Value=ms_fhx4
  Constant4 : Constant  Value=mcp_p_fhx4
  Constant5 : Constant  Value=mcp_s_fhx4
  Constant6 : Constant  Value=mcp_t_fhx4
  Constant7 : Constant  Value=mp_fhx4m
  Constant8 : Constant  Value=hA_p_fhx4
  Constant9 : Constant  Value=hA_s_fhx4
  Demux{,1..5} (6 alike) : Demux
  Demux6 : Demux  Outputs=2
  Divide{,1..16,18..21} (21 alike) : Product  Inputs=***/
  Fuel Heat Exchanger Fuel Temps : Scope  NumInputPorts=5
  Fuel Heat Exchanger Secondary Temps : Scope  NumInputPorts=5
  Fuel Heat Exchanger tube Temps : Scope  NumInputPorts=2
  Minus{,3,7,10,13..15,18..20,23,25,29,33} (14 alike) : Sum
  Minus{1..2,4..6,8..9,11..12,16..17,21..22,24,26..28,30..31,34..35} (21 alike) : Sum  Inputs=+-
  Mux : Mux  Inputs=2
  Mux2 : Mux  Inputs=17
  Mux3 : Mux  Inputs=5
  Mux4 : Mux  Inputs=5
  T_p1 : Integrator  InitialCondition=T0_p_fhx4(1)
  T_p2 : Integrator  InitialCondition=T0_p_fhx4(2)
  "T_p3 " : Integrator  InitialCondition=T0_p_fhx4(3)
  T_p4 : Integrator  InitialCondition=T0_p_fhx4(4)
  T_pm : Integrator  InitialCondition=T0_p_fhx4m
  T_s1 : Integrator  InitialCondition=T0_s_fhx4(1)
  T_s2 : Integrator  InitialCondition=T0_s_fhx4(2)
  T_s3 : Integrator  InitialCondition=T0_s_fhx4(3)
  T_s4 : Integrator  InitialCondition=T0_s_fhx4(4)
  T_t1 : Integrator  InitialCondition=T0_t_fhx4(1)
  T_t2 : Integrator  InitialCondition=T0_t_fhx4(2)
  To Workspace : ToWorkspace  VariableName=Fuel_Heat_Ex_4_Tube_Temps  SaveFormat=Timeseries  SampleTime=-1
  To Workspace2 : ToWorkspace  VariableName=Fuel_Heat_Ex_4_Mux  SaveFormat=Timeseries  SampleTime=-1
  To Workspace3 : ToWorkspace  VariableName=Fuel_Heat_Ex_4_Fuel_Temps  SaveFormat=Timeseries  SampleTime=-1
  To Workspace4 : ToWorkspace  VariableName=Fuel_Heat_Ex_4_Cool_Temps  SaveFormat=Timeseries  SampleTime=-1
  Fuel Exit Temp : Outport
  Coolant Exit Temp : Outport  Port=2
  wires:
  [hA_p_1] -> Divide1/2
  [Wp] -> Divide/2
  [T_p3] -> Minus22/1
  Minus10/1 -> T_p4/1
  Divide3/1 -> Minus3/2
  T_p1/1 -> Minus4/1, [T_p1], Minus1/2, Minus2/2, Minus5/2
  [cool_hA_frac] -> Divide16/1
  Minus25/1 -> T_s4/1
  Demux4/4 -> [mcp_s_4]
  [cool_hA_frac] -> Divide14/1
  Minus9/1 -> Divide6/3
  [Ts_in] -> Minus24/1
  Fuel Heat Transfer Fraction/1 -> [fuel_hA_frac]
  T_s3/1 -> Minus35/2, Minus34/2, Minus27/2, [T_s3], Minus26/1
  [mcp_t_1] -> Divide9/4
  [fuel_flow_frac] -> Divide4/1
  [fuel_hA_frac] -> Divide6/1
  Constant4/1 -> Demux1/1
  Divide18/1 -> Minus33/1
  Demux2/2 -> [hA_p_2]
  [hA_p_1] -> Minus14/1
  [mcp_t_2] -> Divide12/4
  [mcp_t_2] -> Divide11/4
  [hA_s_1] -> Minus20/1
  Minus21/1 -> Divide11/3
  [T_s1] -> Minus21/1
  Minus28/1 -> Divide14/3
  Divide11/1 -> Minus18/2
  Divide7/1 -> Minus10/1
  [hA_p_3] -> Divide6/2
  Minus17/1 -> Divide9/3
  [mcp_p_3] -> Divide6/4
  Divide14/1 -> Minus23/2
  Divide6/1 -> Minus7/2
  [Ws] -> Divide15/2
  [Ws] -> Divide13/2
  Minus15/1 -> Divide10/2
  Minus33/1 -> T_s3/1
  Fuel Flow Fraction/1 -> [fuel_flow_frac]
  [Tf_out] -> Fuel Exit Temp/1
  T_s4/1 -> [Ts_out], Minus26/2, [T_s4]
  Constant7/1 -> [mp_m]
  [mcp_s_3] -> Divide19/4
  Minus30/1 -> Divide15/3
  [T_t1] -> Minus35/1
  Divide8/1 -> Minus10/2
  Divide19/1 -> Minus33/2
  [T_t2] -> Minus12/1
  Minus16/1 -> Divide10/3
  [fuel_hA_frac] -> Divide1/1
  Minus12/1 -> Divide8/3
  [mcp_p_4] -> Divide8/4
  Minus8/1 -> Divide5/3
  "T_p3 "/1 -> Minus11/1, [T_p3], Minus12/2, Minus8/2, Minus9/2
  [fuel_hA_frac] -> Divide8/1
  Demux3/2 -> [ms_2]
  Divide1/1 -> Minus/2
  Minus11/1 -> Divide7/3
  Divide/1 -> Minus/1
  [T_p1] -> Minus17/1
  [cool_flow_frac] -> Divide18/1
  [mcp_s_2] -> Divide16/4
  Demux/4 -> [mp_4]
  Minus4/1 -> Divide2/3
  Divide2/1 -> Minus3/1
  [fuel_flow_frac] -> Divide2/1
  [fuel_hA_frac] -> Divide3/1
  Minus5/1 -> Divide3/3
  Minus35/1 -> Divide19/3
  Demux2/3 -> [hA_p_3]
  [ms_2] -> Divide15/4
  [Wp] -> Divide2/2
  [Tf_in] -> Minus1/1
  Demux3/4 -> [ms_4]
  Divide16/1 -> Minus29/2
  [mp_2] -> Divide2/4
  Demux6/1 -> [mcp_t_1]
  Demux/1 -> [mp_1]
  [cool_flow_frac] -> Divide20/1
  Divide9/1 -> Minus13/1
  Constant6/1 -> Demux6/1
  Constant3/1 -> Demux3/1
  Demux5/2 -> [hA_s_2]
  [hA_s_3] -> Divide19/2
  Demux2/4 -> [hA_p_4]
  [T_t1] -> Minus5/1
  Minus18/1 -> T_t2/1
  [T_t2] -> Minus28/1
  [mcp_t_1] -> Divide10/4
  Minus29/1 -> T_s2/1
  T_t2/1 -> [T_t2], Minus21/2, Minus22/2
  Fuel Inlet Temp/1 -> [Tf_in]
  [Wp] -> Divide7/2
  [Ts_out] -> Coolant Exit Temp/1
  Minus22/1 -> Divide12/3
  [fuel_flow_frac] -> Divide5/1
  [mcp_s_4] -> Divide21/4
  Minus13/1 -> T_t1/1
  [Wp] -> Divide5/2
  Minus3/1 -> T_p2/1
  [mp_3] -> Divide5/4
  Minus2/1 -> Divide1/3
  [cool_hA_frac] -> Divide11/1
  [fuel_flow_frac] -> Divide7/1
  [Ws] -> Divide18/2
  [ms_3] -> Divide18/4
  [T_t1] -> Minus27/1
  Divide21/1 -> Minus25/2
  Minus7/1 -> "T_p3 "/1
  [hA_s_3] -> Minus15/1
  Divide20/1 -> Minus25/1
  T_s1/1 -> Minus31/2, Minus28/2, Minus24/2, [T_s1], Minus30/1
  [hA_s_2] -> Divide16/2
  [fuel_hA_frac] -> Divide9/1
  Minus6/1 -> Divide4/3
  [hA_s_4] -> Minus15/2
  Divide10/1 -> Minus13/2
  [hA_p_4] -> Divide8/2
  T_s2/1 -> Minus34/1, Minus30/2, [T_s2]
  [cool_flow_frac] -> Divide13/1
  [Wp] -> Divide4/2
  [hA_p_3] -> Minus19/1
  [cool_flow_frac] -> Divide15/1
  Minus31/1 -> Divide16/3
  [T_s3] -> Minus16/1
  Minus27/1 -> Divide21/3
  [cool_hA_frac] -> Divide21/1
  Demux1/3 -> [mcp_p_3]
  Constant1/1 -> Demux/1
  Demux5/4 -> [hA_s_4]
  [cool_hA_frac] -> Divide10/1
  Divide12/1 -> Minus18/1
  Demux3/1 -> [ms_1]
  Demux/2 -> [mp_2]
  [mp_1] -> Divide/4
  Demux4/1 -> [mcp_s_1]
  T_p4/1 -> [Tf_out], [T_p4], Minus11/2
  [T_t2] -> Minus31/1
  Demux2/1 -> [hA_p_1]
  Divide4/1 -> T_pm/1
  [hA_s_4] -> Divide21/2
  [mp_4] -> Divide7/4
  Minus1/1 -> Divide/3
  Demux/3 -> [mp_3]
  Minus19/1 -> Divide12/2
  Minus24/1 -> Divide13/3
  [T_t1] -> Minus2/1
  Demux1/4 -> [mcp_p_4]
  [ms_1] -> Divide13/4
  Demux3/3 -> [ms_3]
  [fuel_flow_frac] -> Divide/1
  Demux6/2 -> [mcp_t_2]
  Constant2/1 -> [Ws]
  Minus/1 -> T_p1/1
  [hA_s_2] -> Minus20/2
  [hA_p_2] -> Divide3/2
  Coolant Flow Fraction/1 -> [cool_flow_frac]
  Minus23/1 -> T_s1/1
  Divide15/1 -> Minus29/1
  [ms_4] -> Divide20/4
  [mcp_p_1] -> Divide1/4
  Coolant Heat Transfer Fraction/1 -> [cool_hA_frac]
  T_pm/1 -> [T_pm], Minus6/2, Minus8/1
  [T_t2] -> Minus9/1
  Divide13/1 -> Minus23/1
  Constant9/1 -> Demux5/1
  [Ws] -> Divide20/2
  T_t1/1 -> [T_t1], Minus16/2, Minus17/2
  Demux5/1 -> [hA_s_1]
  Minus26/1 -> Divide20/3
  [mcp_p_2] -> Divide3/4
  [cool_hA_frac] -> Divide19/1
  Minus34/1 -> Divide18/3
  Constant/1 -> [Wp]
  [mp_m] -> Divide4/4
  [hA_p_4] -> Minus19/2
  Demux4/3 -> [mcp_s_3]
  Minus20/1 -> Divide11/2
  Divide5/1 -> Minus7/1
  Demux1/2 -> [mcp_p_2]
  Coolant Inlet Temp/1 -> [Ts_in]
  [mcp_s_1] -> Divide14/4
  Demux4/2 -> [mcp_s_2]
  T_p2/1 -> [T_p2], Minus4/2, Minus6/1
  Constant5/1 -> Demux4/1
  [fuel_hA_frac] -> Divide12/1
  Demux5/3 -> [hA_s_3]
  Minus14/1 -> Divide9/2
  [hA_p_2] -> Minus14/2
  Constant8/1 -> Demux2/1
  [hA_s_1] -> Divide14/2
  Demux1/1 -> [mcp_p_1]
  [T_s2] -> Mux4/3, Fuel Heat Exchanger Secondary Temps/3, Mux2/11
  [T_pm] -> Mux2/5
  [T_t2] -> Mux2/9, Mux/2, Fuel Heat Exchanger tube Temps/2
  [cool_hA_frac] -> Mux2/17
  [T_s1] -> Mux4/2, Fuel Heat Exchanger Secondary Temps/2, Mux2/10
  [T_s4] -> Fuel Heat Exchanger Secondary Temps/5, Mux4/5, Mux2/13
  [cool_flow_frac] -> Mux2/16
  [Tf_in] -> Fuel Heat Exchanger Fuel Temps/1, Mux3/1, Mux2/1
  [Ts_in] -> Mux4/1, Fuel Heat Exchanger Secondary Temps/1, Mux2/2
  [T_t1] -> Mux/1, Fuel Heat Exchanger tube Temps/1, Mux2/8
  [T_s3] -> Mux4/4, Fuel Heat Exchanger Secondary Temps/4, Mux2/12
  [T_p2] -> Mux2/4, Mux3/3, Fuel Heat Exchanger Fuel Temps/3
  [T_p4] -> Mux3/5, Fuel Heat Exchanger Fuel Temps/5, Mux2/7
  Mux2/1 -> To Workspace2/1
  [fuel_hA_frac] -> Mux2/15
  [T_p3] -> Mux3/4, Fuel Heat Exchanger Fuel Temps/4, Mux2/6
  Mux4/1 -> To Workspace4/1
  [fuel_flow_frac] -> Mux2/14
  [T_p1] -> Mux3/2, Fuel Heat Exchanger Fuel Temps/2, Mux2/3
  Mux/1 -> To Workspace/1
  Mux3/1 -> To Workspace3/1
